simulink model "Vehicle_model_with_controllers_in_continuous_system_V01"  (R2026a)
settings: Solver=VariableStepAuto  StopTime=inf  RelTol=1e-6
InitFcn:
  | run('Vehicle_parameters_values_V1_MIL.m')
undefined symbols (not defined in the file): Finaldrive, Transmission, Vehicle
libraries: slpidlib x2
(part 1 of 2)
settings Model: PacingRate=0.500000  Creator=irfan  LastModifiedBy=irfan
settings SolverCC: ShapePreserveControl=EnableAll  ZeroCrossControl=EnableAll  ZeroCrossAlgorithm=Adaptive  MinimalZcImpactIntegration=on
settings DebuggingCC: ReadBeforeWriteMsg=DisableAll  WriteAfterWriteMsg=DisableAll  WriteAfterReadMsg=DisableAll  MultiTaskDSMMsg=none
settings SFSimCC: SFSimEcho=off

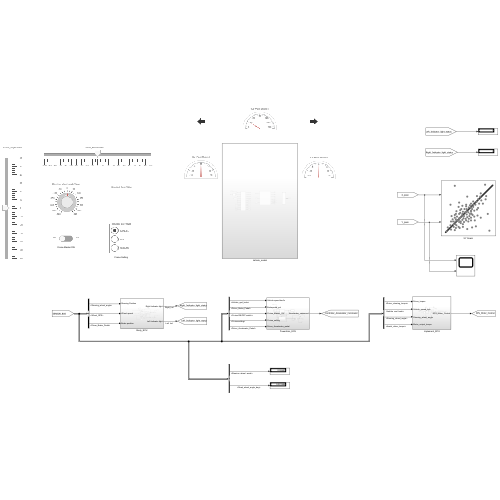
[thumbnail: Simulink's stored preview of the top-level diagram]
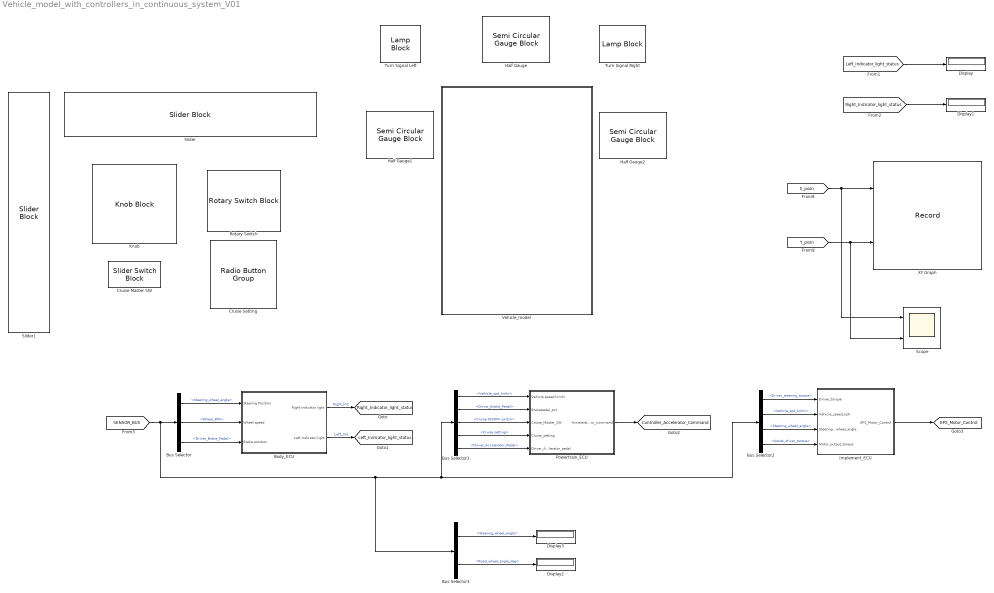
== system Vehicle_model_with_controllers_in_continuous_system_V01 ==
  Body_ECU : Subsystem
  Bus Selector : BusSelector  OutputSignals=Steering_wheel_angle,Wheel_RPS,Driver_Brake_Pedal
  Bus Selector1 : BusSelector  OutputSignals=Vehicle_spd_kmhr,Driver_Brake_Pedal,Cruise ON/OFF switch,Cruise setting,Driver_Accelerator_Pedal
  Bus Selector2 : BusSelector  OutputSignals=Driver_steering_torque,Vehicle_spd_kmhr,Steering_wheel_angle,Assist_driver_torque
  Bus Selector3 : BusSelector  OutputSignals=Steering_wheel_angle,Road_wheel_angle_deg
  Cruise Master SW : SliderSwitchBlock  LabelPosition=Hide
  Cruise Setting : RadioButtonGroup  LabelPosition=Hide  SelectedLabel=CANCEL  ButtonGroupName=CRUISE_SETTING
  Display{,1..3} (4 alike) : Display
  Half Gauge : SemiCircularGaugeBlock  ScaleMax=180  FontColor=[0.0, 0.0, 0.0]
  Half Gauge1 : SemiCircularGaugeBlock  ScaleMin=-15  ScaleMax=15  TickInterval=5  FontColor=[0.0, 0.0, 0.0]
  Half Gauge2 : SemiCircularGaugeBlock  ScaleMin=-15  ScaleMax=15  TickInterval=5  FontColor=[0.0, 0.0, 0.0]
  Implement_ECU : Subsystem
  Knob : KnobBlock  ScaleMin=-540  ScaleMax=540  TickInterval=90
  Powertrain_ECU : Subsystem
  Rotary Switch : RotarySwitchBlock
  Scope : Scope  NumInputPorts=2
      settings: ActiveDisplayYMinimum=-16.839005262411046  ActiveDisplayYMaximum=22.945762776973872  DataLoggingVariableName=ScopeData55
  Slider : SliderBlock  ScaleMin=-100  TickInterval=10
  Slider1 : SliderBlock  ScaleMin=-60  ScaleMax=60  TickInterval=10
  Turn Signal Left : LampBlock  LabelPosition=Hide  DefaultColor=[192.0, 192.0, 192.0]  Icon=TurnSignalLeft
  Turn Signal Right : LampBlock  LabelPosition=Hide  DefaultColor=[192.0, 192.0, 192.0]  Icon=TurnSignalRight
  Vehicle_model : Subsystem
  XY Graph : Record  NumPorts=2.0  FileSettingsInternal="{\"entries\":[{\"content\":{\"excelSettings\":{\"content\":{},\"type\":\"Streamout.ExcelSettings\"},\"parquetSettings\":{\"content\":{},\"type\":\"Streamout.ParquetSettings\"}},\"type\":\"Streamout.FileSettingStorage\",\"uuid\":\"\"}],\"packageUris\":[\"http:\\/\\/schema.mathworks.com\\/mf0\\/streamout_blocks\\/R2020a\"],\"version\":\"1.0\"}"  FrameSettings=[0, 0]  Layout=[1 1]  SignalsInternal="{\"entries\":[{\"content\":{\"signals\":[{\"content\":{\"blockPath\":[],\"dimensions\":[1],\"domain\":\"\",\"lineColor\":\"#a2142f\",\"plots\":[ 1 ],\"port\":1,\"sid\":[\"\"],\"signalID\":1,\"signalName\":\"From8\"},\"type\":\"RecordBlkView.Signal\",\"uuid\":\"\"},{\"content\":{\"blockPath\":[],\"dimensions\":[1],\"domain\":\"\",\"lineColor\":\"#139fff\",\"plots\":[ 1 ],\"port\":2,\"sid\":[\"\"],\"signalID\":2,\"signalName\":\"From9\"},\"type\":\"RecordBlkView.Signal\",\"uuid\":\"\"},{\"content\":{\"blockPath\":[],\"dimensions\":[1],\"domain\":\"\",\"lineColor\":\"#77ac30\",\"lineWidth\":2,\"sid\":[\"\"],\"signalID\":3,\"signalName\":\"Grade_angle:Value\"},\"type\":\"RecordBlkView.Signal\",\"uuid\":\"\"},{\"content\":{\"blockPath\":[],\"dimensions\":[1],\"domain\":\"\",\"lineColor\":\"#4dbeee\",\"lineWidth\":2,\"sid\":[\"\"],\"signalID\":4,\"signalName\":\"CruiseMasterSW:Value\"},\"type\":\"RecordBlkView.Signal\",\"uuid\":\"\"},{\"content\":{\"blockPath\":[],\"dimensions\":[1],\"domain\":\"\",\"lineColor\":\"#a2142f\",\"lineWidth\":2,\"sid\":[\"\"],\"signalID\":5,\"signalName\":\"Cruisesetting:Value\"},\"type\":\"RecordBlkView.Signal\",\"uuid\":\"\"},{\"content\":{\"blockPath\":[],\"dimensions\":[1],\"domain\":\"\",\"lineColor\":\"#139fff\",\"lineWidth\":2,\"sid\":[\"\"],\"signalID\":6,\"signalName\":\"Driver_Pedal:Value\"},\"type\":\"RecordBlkView.Signal\",\"uuid\":\"\"},{\"content\":{\"blockPath\":[],\"dimensions\":[1],\"domain\":\"\",\"lineColor\":\"#ff6929\",\"lineWidth\":2,\"sid\":[\"\"],\"signalID\":7,\"signalName\":\"Selected_Gear:Value\"},\"type\":\"RecordBlkView.Signal\",\"uuid\":\"\"},{\"content\":{\"blockPath\":[],\"dimensions\":[1],\"domain\":\"\",\"lineColor\":\"#b746ff\",\"lineWidth\":2,\"sid\":[\"\"],\"signalID\":8,\"signalName\":\"Steering_wheel_angle:Value\"},\"type\":\"RecordBlkView.Signal\",\"uuid\":\"\"}]},\"type\":\"RecordBlkView.InputSignals\",\"uuid\":\"\"}],\"packageUris\":[\"http:\\/\\/schema.mathworks.com\\/mf0\\/streamout_blocks\\/R2020a\"],\"version\":\"1.0\"}"  VisualizationBindings="{\"xyplotplugin\":{\"info\":[{\"series\":[{\"bindingParametersList\":[{\"parameter\":\"X-Axis\",\"signalID\":1,\"signalName\":\"From8\"},{\"parameter\":\"Y-Axis\",\"signalID\":2,\"signalName\":\"From9\"}],\"seriesID\":0}],\"subplotID\":1}]}}"  CompatibilityTag=XY
  tag scope: Controller_Accelerator_Command=global, EPS_Motor_Control=global, Left_Indicator_light_status=global, Right_Indicator_light_status=global
  wires:
  Bus Selector/1 -> Body_ECU/1(Steering Position)  "<Steering_wheel_angle>"
  Bus Selector/3 -> Body_ECU/3(Brake position)  "<Driver_Brake_Pedal>"
  Body_ECU/1(Right Indicator light) -> [Right_Indicator_light_status]  "Right_Ind"
  Body_ECU/2(Left Indicator light) -> [Left_Indicator_light_status]  "Left_Ind"
  Bus Selector/2 -> Body_ECU/2(Wheel speed)  "<Wheel_RPS>"
  Bus Selector1/1 -> Powertrain_ECU/1(Vehicle speed km/hr)  "<Vehicle_spd_kmhr>"
  Bus Selector1/2 -> Powertrain_ECU/2(Brakepedal_pct)  "<Driver_Brake_Pedal>"
  Bus Selector1/3 -> Powertrain_ECU/3(Cruise_Master_SW)  "<Cruise ON/OFF switch>"
  Bus Selector1/4 -> Powertrain_ECU/4(Cruise_setting)  "<Cruise setting>"
  Bus Selector1/5 -> Powertrain_ECU/5(Driver_Accelerator_pedal)  "<Driver_Accelerator_Pedal>"
  Powertrain_ECU/1(Accelerator_command) -> [Controller_Accelerator_Command]
  Bus Selector2/1 -> Implement_ECU/1(Driver_torque)  "<Driver_steering_torque>"
  Bus Selector2/2 -> Implement_ECU/2(Vehicle_speed_kph)  "<Vehicle_spd_kmhr>"
  Bus Selector2/3 -> Implement_ECU/3(Steering_wheel_angle)  "<Steering_wheel_angle>"
  Bus Selector2/4 -> Implement_ECU/4(Motor_output_torque)  "<Assist_driver_torque>"
  Implement_ECU/1(EPS_Motor_Control) -> [EPS_Motor_Control]
  [X_posn] -> Scope/1, XY Graph/1
  [Y_posn] -> Scope/2, XY Graph/2
  [Left_Indicator_light_status] -> Display/1
  [Right_Indicator_light_status] -> Display1/1
  [SENSOR_BUS] -> Bus Selector3/1, Bus Selector2/1, Bus Selector1/1, Bus Selector/1
  Bus Selector3/2 -> Display2/1  "<Road_wheel_angle_deg>"
  Bus Selector3/1 -> Display3/1  "<Steering_wheel_angle>"

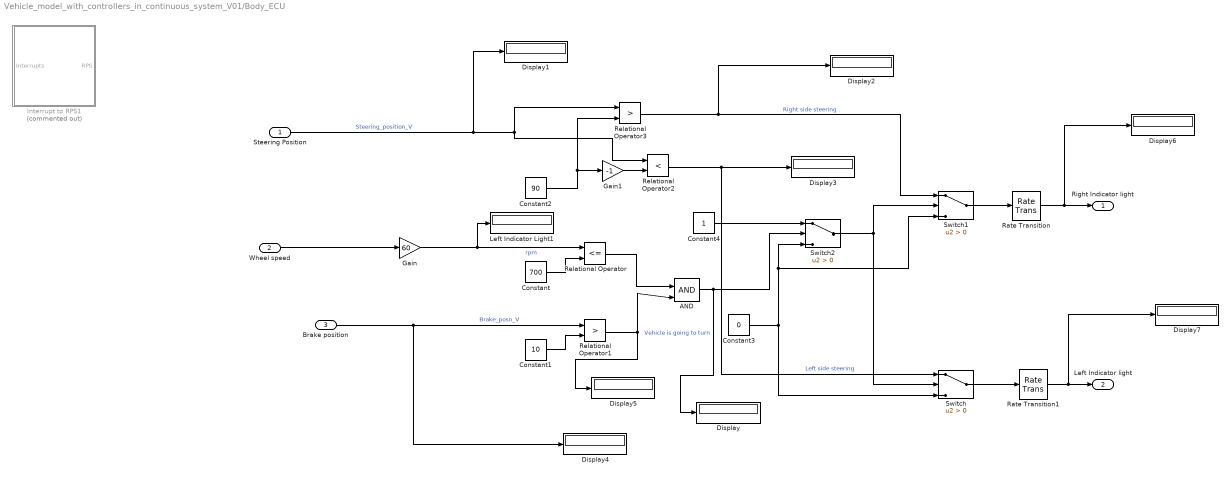
== system Vehicle_model_with_controllers_in_continuous_system_V01/Body_ECU ==
  Steering Position : Inport  OutDataTypeStr=single  PortDimensions=1
  Wheel speed : Inport  Port=2  OutDataTypeStr=double  PortDimensions=1
  Brake position : Inport  Port=3  OutDataTypeStr=double  PortDimensions=1
  AND : Logic  IconShape=distinctive  AllPortsSameDT=off  OutDataTypeStr=boolean
  Constant : Constant  Value=700
  Constant1 : Constant  Value=10
  Constant2 : Constant  Value=90
  Constant3 : Constant  Value=0
  Constant4 : Constant
  Display{,1..7} (8 alike) : Display
  Gain : Gain  Gain=60
  Gain1 : Gain  Gain=-1
  Interrupt to RPS1 : Subsystem  Commented=on
  Left Indicator Light1 : Display
  Rate Transition : RateTransition
  Rate Transition1 : RateTransition
  Relational Operator : RelationalOperator  Operator=<=  OutDataTypeStr=boolean  RndMeth=Simplest  InputSameDT=off
  Relational Operator1 : RelationalOperator  Operator=>  OutDataTypeStr=boolean  RndMeth=Simplest  InputSameDT=off
  Relational Operator2 : RelationalOperator  Operator=<  OutDataTypeStr=boolean  RndMeth=Simplest  InputSameDT=off
  Relational Operator3 : RelationalOperator  Operator=>  OutDataTypeStr=boolean  RndMeth=Simplest  InputSameDT=off
  Switch : Switch  Criteria=u2 > Threshold  SaturateOnIntegerOverflow=off  InputSameDT=off
  Switch1 : Switch  Criteria=u2 > Threshold  SaturateOnIntegerOverflow=off  InputSameDT=off
  Switch2 : Switch  Criteria=u2 > Threshold  SaturateOnIntegerOverflow=off  InputSameDT=off
  Right Indicator light : Outport  OutDataTypeStr=double  PortDimensions=1  SampleTime=[0,1]
  Left Indicator light : Outport  Port=2  OutDataTypeStr=double  PortDimensions=1  SampleTime=[0,1]
  wires:
  Rate Transition1/1 -> Display7/1, Left Indicator light/1
  Relational Operator/1 -> AND/1
  Rate Transition/1 -> Display6/1, Right Indicator light/1
  Constant1/1 -> Relational Operator1/2
  Constant4/1 -> Switch2/1
  Gain/1 -> Relational Operator/1, Left Indicator Light1/1  "rpm"
  Switch2/1 -> Switch/2, Switch1/2
  Constant/1 -> Relational Operator/2
  AND/1 -> Display/1, Switch2/2  "Vehicle is going to turn"
  Switch/1 -> Rate Transition1/1
  Constant2/1 -> Gain1/1, Relational Operator3/2
  Relational Operator1/1 -> AND/2, Display5/1
  Steering Position/1 -> Display1/1, Relational Operator3/1, Relational Operator2/1  "Steering_position_V"
  Brake position/1 -> Display4/1, Relational Operator1/1  "Brake_posn_V"
  Constant3/1 -> Switch/3, Switch1/3, Switch2/3
  Relational Operator2/1 -> Switch/1, Display3/1  "Left side steering"
  Relational Operator3/1 -> Display2/1, Switch1/1  "Right side steering"
  Switch1/1 -> Rate Transition/1
  Gain1/1 -> Relational Operator2/2
  Wheel speed/1 -> Gain/1

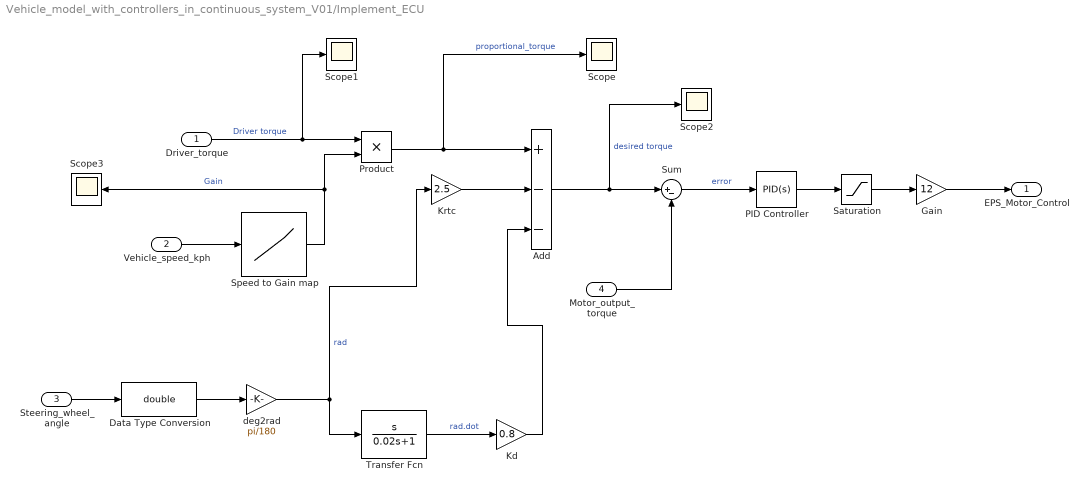
== system Vehicle_model_with_controllers_in_continuous_system_V01/Implement_ECU ==
  Driver_torque : Inport
  Vehicle_speed_kph : Inport  Port=2
  Steering_wheel_angle : Inport  Port=3
  Motor_output_torque : Inport  Port=4
  Add : Sum  Inputs=+--
  Data Type Conversion : DataTypeConversion  OutDataTypeStr=double  SaturateOnIntegerOverflow=off  RndMeth=Floor
  Gain : Gain  Gain=12
  Kd : Gain  Gain=0.8
  Krtc : Gain  Gain=2.5
  PID Controller : slpidlib/PID Controller  Controller=PID  Form=Parallel  TimeDomain=Continuous-time  UseExternalTs=off  SampleTime=-1  IntegratorMethod=Forward Euler  FilterMethod=Forward Euler  ControllerParametersSource=internal  P=1  I=5  UseKiTs=off  D=0  UseExternalDerivativeSource=off  N=100  UseFilter=on  TunerSelectOption=Transfer Function Based (PID Tuner App)  InitialConditionSource=internal  InitialConditionForIntegrator=0  InitialConditionForFilter=0  DifferentiatorICPrevScaledInput=0  ExternalReset=none  TrackingMode=off  Kt=1  LimitOutput=off  SatLimitsSource=internal  UpperSaturationLimit=inf  LowerSaturationLimit=-inf  LinearizeAsGain=on  AntiWindupMode=none  Kb=1  LimitIntegrator=off  UpperIntegratorSaturationLimit=inf  LowerIntegratorSaturationLimit=-inf  POutMin=[]  POutMax=[]  IOutMin=[]  IOutMax=[]  DOutMin=[]  DOutMax=[]  NOutMin=[]  NOutMax=[]  SumOutMin=[]  SumOutMax=[]  SaturationOutMin=[]  SaturationOutMax=[]  PParamMin=[]  PParamMax=[]  IParamMin=[]  IParamMax=[]  DParamMin=[]  DParamMax=[]  NParamMin=[]  NParamMax=[]  KbParamMin=[]  KbParamMax=[]  KtParamMin=[]  KtParamMax=[]  KbOutMin=[]  KbOutMax=[]  KtOutMin=[]  KtOutMax=[]  IntegratorOutMin=[]  IntegratorOutMax=[]  FilterOutMin=[]  FilterOutMax=[]  SumI1OutMin=[]  SumI1OutMax=[]  SumI2OutMin=[]  SumI2OutMax=[]  SumI3OutMin=[]  SumI3OutMax=[]  SumI4OutMin=[]  SumI4OutMax=[]  SumDOutMin=[]  SumDOutMax=[]  DifferentiatorOutMin=[]  DifferentiatorOutMax=[]  FilterDiffOutCoefMin=[]  FilterDiffOutCoefMax=[]  ReciprocalOutMin=[]  ReciprocalOutMax=[]  SumDenOutMin=[]  SumDenOutMax=[]  SumNumOutMin=[]  SumNumOutMax=[]  DivideOutMin=[]  DivideOutMax=[]  UdiffTsProdOutMin=[]  UdiffTsProdOutMax=[]  NTsProdOutMin=[]  NTsProdOutMax=[]  UintegralTsProdOutMin=[]  UintegralTsProdOutMax=[]  UngainTsProdOutMin=[]  UngainTsProdOutMax=[]  ClampingZeroOutDataTypeStr=Inherit: Inherit via back propagation  ClampingZeroOutMin=[]  ClampingZeroOutMax=[]  FilterDenConstantOutDataTypeStr=Inherit: Inherit via back propagation  FilterDenConstantOutMin=[]  FilterDenConstantOutMax=[]  PCopyOutDataTypeStr=Inherit: Inherit via back propagation  PCopyOutMin=[]  PCopyOutMax=[]  NCopyOutDataTypeStr=Inherit: Inherit via back propagation  NCopyOutMin=[]  NCopyOutMax=[]  IntegratorContinuousStateAttributes=''  IntegratorStateMustResolveToSignalObject=off  IntegratorRTWStateStorageClass=Auto  FilterContinuousStateAttributes=''  FilterStateMustResolveToSignalObject=off  FilterRTWStateStorageClass=Auto  ParallelPVariant=InternalParameters  IdealPVariant=Disabled  IVariant=InternalParameters  DVariant=InternalParameters  IntegratorVariant=Continuous  SatVariant=Disabled  AWVariant=Passthrough  PCopyVariant=Disabled  TRVariant=Disabled  FdbkBlocksVariant=Forward  IdealPFdbkVariant=Disabled  SatFdbkVariant=Disabled  DerivativeFilterVariant=ContFilter  NVariant=InternalParameters  NCopyVariant=Disabled  FilterICVariant=InternalICsFilter  IntegratorICVariant=InternalICs  ExternalResetVariant=Disabled  TRSumVariant=Passthrough  SumFdbkVariant=Disabled  SumVariant=Sum_PID  TsampFilterVariant=InternalTs  TsampNgainVariant=Passthrough  TsampIntegralVariant=Disabled_SignalSpec  ExternalSaturationOutDataTypeStr=Inherit: Same as second input  DerivativeSourceVariant=ErrorSignal  PreIntVariant=InternalPreInt
  Product : Product
  Saturation : Saturate  UpperLimit=1  LowerLimit=0
  Scope{,1..3} (4 alike) : Scope
      Scope settings: DataLoggingVariableName=ScopeData9
      Scope1 settings: ActiveDisplayYMinimum=33.050124587675704  ActiveDisplayYMaximum=33.050574191834883  DataLoggingVariableName=ScopeData10
      Scope2 settings: ActiveDisplayYMinimum=13.852646360753944  ActiveDisplayYMaximum=13.860007449671043  DataLoggingVariableName=ScopeData11
      Scope3 settings: ActiveDisplayYMinimum=-1  ActiveDisplayYMaximum=1  DataLoggingVariableName=ScopeData12
  Speed to Gain map : Lookup_n-D  NumberOfTableDimensions=1  BreakpointsForDimension1=Vehicle.speedvalues  Table=Vehicle.torquegains  InternalRulePriority=Speed  RndMeth=Simplest
  Sum : Sum  Inputs=|+-
  Transfer Fcn : TransferFcn  Numerator=[1 0]  Denominator=[0.02 1]
  deg2rad : Gain  Gain=pi/180
  EPS_Motor_Control : Outport
  wires:
  Speed to Gain map/1 -> Product/2, Scope3/1  "Gain"
  Sum/1 -> PID Controller/1  "error"
  Product/1 -> Scope/1, Add/1  "proportional_torque"
  Driver_torque/1 -> Scope1/1, Product/1  "Driver torque"
  Vehicle_speed_kph/1 -> Speed to Gain map/1
  PID Controller/1 -> Saturation/1
  Motor_output_torque/1 -> Sum/2
  Saturation/1 -> Gain/1
  Gain/1 -> EPS_Motor_Control/1
  Krtc/1 -> Add/2
  Steering_wheel_angle/1 -> Data Type Conversion/1
  deg2rad/1 -> Transfer Fcn/1, Krtc/1  "rad"
  Transfer Fcn/1 -> Kd/1  "rad.dot"
  Add/1 -> Scope2/1, Sum/1  "desired torque"
  Kd/1 -> Add/3
  Data Type Conversion/1 -> deg2rad/1

== system Vehicle_model_with_controllers_in_continuous_system_V01/Powertrain_ECU ==
  Vehicle speed km/hr : Inport
  Brakepedal_pct : Inport  Port=2
  Cruise_Master_SW : Inport  Port=3
  Cruise_setting : Inport  Port=4
  Driver_Accelerator_pedal : Inport  Port=5
  Chart : Stateflow chart  TreatAsAtomicUnit=on
  Display : Display
  Display1 : Display
  Display2 : Display
  Enabled Subsystem : Subsystem  TreatAsAtomicUnit=on
  Scope : Scope
      settings: ActiveDisplayYMinimum=-1  ActiveDisplayYMaximum=1  DataLoggingVariableName=ScopeData6
  Scope1 : Scope
      settings: ActiveDisplayYMinimum=-5.6388294949677089  ActiveDisplayYMaximum=36.997696709911374  DataLoggingVariableName=ScopeData7
  Switch : Switch  Criteria=u2 > Threshold  SaturateOnIntegerOverflow=off  InputSameDT=off
  Accelerator_command : Outport
  wires:
  Chart/1(Set_spd) -> Enabled Subsystem/2(Set_spd), Display/1
  Vehicle speed km/hr/1 -> Chart/3(Vehicle_spd), Enabled Subsystem/1(Vehicle speed km/hr)
  Cruise_Master_SW/1 -> Chart/4(Cruise_Master_SW)
  Brakepedal_pct/1 -> Chart/2(Brk_pdl)
  Enabled Subsystem/1(CruiseAccelPedal_pct) -> Scope/1, Switch/1
  Cruise_setting/1 -> Chart/1(Cr_St)
  Chart/2(Cruise_enable) -> Display1/1, Enabled Subsystem/Enable, Enabled Subsystem/3(CruiseEnable), Switch/2
  Driver_Accelerator_pedal/1 -> Switch/3
  Switch/1 -> Scope1/1, Display2/1, Accelerator_command/1

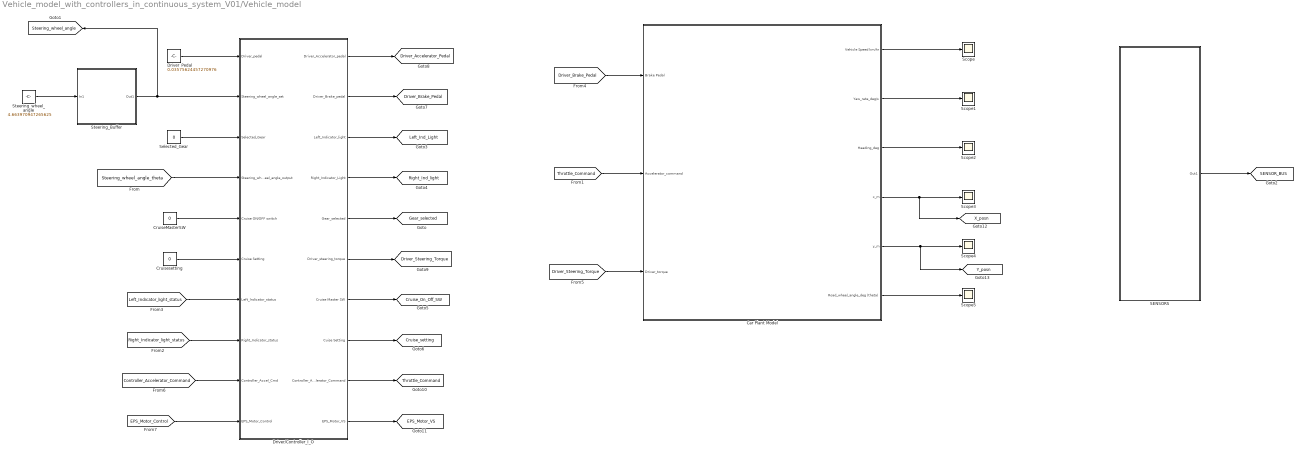
== system Vehicle_model_with_controllers_in_continuous_system_V01/Vehicle_model ==
  Car Plant Model : Subsystem
  CruiseMasterSW : Constant  Value=0
  Cruisesetting : Constant  Value=0
  Driver/Controller_I_O : Subsystem
  Driver_Pedal : Constant  Value=0.03575624457270976
  SENSORS : Subsystem
  Scope{,1..5} (6 alike) : Scope
      Scope settings: ActiveDisplayYMinimum=52.703316874102136  ActiveDisplayYMaximum=58.921674606812623
      Scope2 settings: DataLoggingVariableName=ScopeData2
      Scope3 settings: DataLoggingVariableName=ScopeData3
      Scope4 settings: DataLoggingVariableName=ScopeData4
      Scope5 settings: ActiveDisplayYMinimum=-229.29250394050729  ActiveDisplayYMaximum=178.246522265426  DataLoggingVariableName=ScopeData5
  Selected_Gear : Constant  Value=0
  Steering_Buffer : Subsystem
  Steering_wheel_angle : Constant  Value=4.663970947265625
  tag scope: Cruise_On_Off_SW=global, Cruise_setting=global, Driver_Accelerator_Pedal=global, Driver_Brake_Pedal=global, Driver_Steering_Torque=global, EPS_Motor_VS=global, Gear_selected=global, Left_Ind_Light=global, Right_Ind_light=global, SENSOR_BUS=global, Steering_wheel_angle=global, Throttle_Command=global, X_posn=global, Y_posn=global
  wires:
  Selected_Gear/1 -> Driver/Controller_I_O/3(Selected_Gear)
  Driver_Pedal/1 -> Driver/Controller_I_O/1(Driver_pedal)
  [Steering_wheel_angle_theta] -> Driver/Controller_I_O/4(Steering_wheel_angle_output)
  Driver/Controller_I_O/5(Gear_selected) -> [Gear_selected]
  SENSORS/1(Out1) -> [SENSOR_BUS]
  Driver/Controller_I_O/3(Left_Indicator_light) -> [Left_Ind_Light]
  Driver/Controller_I_O/4(Right_Indicator_Light) -> [Right_Ind_light]
  Cruisesetting/1 -> Driver/Controller_I_O/6(Cruise Setting)
  CruiseMasterSW/1 -> Driver/Controller_I_O/5(Cruise ON/OFF switch)
  Car Plant Model/1(Vehicle Speed km/hr) -> Scope/1
  Car Plant Model/2(Yaw_rate_deg/s) -> Scope1/1
  Car Plant Model/3(Heading_deg) -> Scope2/1
  Car Plant Model/4(x_m) -> [X_posn], Scope3/1
  Car Plant Model/5(y_m) -> [Y_posn], Scope4/1
  Car Plant Model/6(Road_wheel_angle_deg (theta)) -> Scope5/1
  [Right_Indicator_light_status] -> Driver/Controller_I_O/8(Right_Indicator_status)
  [Left_Indicator_light_status] -> Driver/Controller_I_O/7(Left_lndicator_status)
  Driver/Controller_I_O/7(Cruise Master SW) -> [Cruise_On_Off_SW]
  Driver/Controller_I_O/8(Cuise Setting) -> [Cruise_setting]
  Driver/Controller_I_O/2(Driver_Brake_pedal) -> [Driver_Brake_Pedal]
  [Driver_Brake_Pedal] -> Car Plant Model/1(Brake Pedal)
  Driver/Controller_I_O/1(Driver_Accelerator_pedal) -> [Driver_Accelerator_Pedal]
  Driver/Controller_I_O/6(Driver_steering_torque) -> [Driver_Steering_Torque]
  [Driver_Steering_Torque] -> Car Plant Model/3(Driver_torque)
  [Controller_Accelerator_Command] -> Driver/Controller_I_O/9(Controller_Accel_Cmd)
  Driver/Controller_I_O/9(Controller_Accelerator_Command) -> [Throttle_Command]
  [EPS_Motor_Control] -> Driver/Controller_I_O/10(EPS_Motor_Control)
  Driver/Controller_I_O/10(EPS_Motor_VS) -> [EPS_Motor_VS]
  [Throttle_Command] -> Car Plant Model/2(Accelerator_command)
  Steering_wheel_angle/1 -> Steering_Buffer/1(In1)
  Steering_Buffer/1(Out1) -> [Steering_wheel_angle], Driver/Controller_I_O/2(Steering_wheel_angle_set)

== system Vehicle_model_with_controllers_in_continuous_system_V01/Body_ECU/Interrupt to RPS1 ==
  Interrupts : Inport
  Data Store Memory : DataStoreMemory  DataStoreName=Count  WriteAfterWriteMsg=warning  ShowAdditionalParam=off
  Pulse Generator : DiscretePulseGenerator  PulseType=Time based  Period=1.1  PulseWidth=10
  Scope3 : Scope
      settings: ActiveDisplayYMinimum=-0.12499999999999997  ActiveDisplayYMaximum=1.125  DataLoggingVariableName=ScopeData2
  Triggered Subsystem : Subsystem  TreatAsAtomicUnit=on
  Triggered Subsystem1 : Subsystem  TreatAsAtomicUnit=on
  RPS : Outport
  wires:
  Interrupts/1 -> Triggered Subsystem/Trigger
  Pulse Generator/1 -> Scope3/1, Triggered Subsystem1/Trigger
  Triggered Subsystem/1(RPS) -> RPS/1

== system Vehicle_model_with_controllers_in_continuous_system_V01/Powertrain_ECU/Enabled Subsystem ==
  Vehicle speed km/hr : Inport
  Set_spd : Inport  Port=2
  CruiseEnable : Inport  Port=3
  Enable : EnablePort  StatesWhenEnabling=reset
  Dead Zone : DeadZone
  NOT : Logic  Operator=NOT  IconShape=distinctive  AllPortsSameDT=off  OutDataTypeStr=boolean
  PID Controller : slpidlib/PID Controller  Controller=PID  Form=Parallel  TimeDomain=Continuous-time  UseExternalTs=off  SampleTime=-1  IntegratorMethod=Forward Euler  FilterMethod=Forward Euler  ControllerParametersSource=internal  P=1  I=0.5  UseKiTs=off  D=0  UseExternalDerivativeSource=off  N=100  UseFilter=on  TunerSelectOption=Transfer Function Based (PID Tuner App)  InitialConditionSource=internal  InitialConditionForIntegrator=0  InitialConditionForFilter=0  DifferentiatorICPrevScaledInput=0  ExternalReset=rising  TrackingMode=off  Kt=1  LimitOutput=on  SatLimitsSource=internal  UpperSaturationLimit=100  LowerSaturationLimit=0  LinearizeAsGain=on  AntiWindupMode=back-calculation  Kb=1  LimitIntegrator=off  UpperIntegratorSaturationLimit=inf  LowerIntegratorSaturationLimit=-inf  POutMin=[]  POutMax=[]  IOutMin=[]  IOutMax=[]  DOutMin=[]  DOutMax=[]  NOutMin=[]  NOutMax=[]  SumOutMin=[]  SumOutMax=[]  SaturationOutMin=[]  SaturationOutMax=[]  PParamMin=[]  PParamMax=[]  IParamMin=[]  IParamMax=[]  DParamMin=[]  DParamMax=[]  NParamMin=[]  NParamMax=[]  KbParamMin=[]  KbParamMax=[]  KtParamMin=[]  KtParamMax=[]  KbOutMin=[]  KbOutMax=[]  KtOutMin=[]  KtOutMax=[]  IntegratorOutMin=[]  IntegratorOutMax=[]  FilterOutMin=[]  FilterOutMax=[]  SumI1OutMin=[]  SumI1OutMax=[]  SumI2OutMin=[]  SumI2OutMax=[]  SumI3OutMin=[]  SumI3OutMax=[]  SumI4OutMin=[]  SumI4OutMax=[]  SumDOutMin=[]  SumDOutMax=[]  DifferentiatorOutMin=[]  DifferentiatorOutMax=[]  FilterDiffOutCoefMin=[]  FilterDiffOutCoefMax=[]  ReciprocalOutMin=[]  ReciprocalOutMax=[]  SumDenOutMin=[]  SumDenOutMax=[]  SumNumOutMin=[]  SumNumOutMax=[]  DivideOutMin=[]  DivideOutMax=[]  UdiffTsProdOutMin=[]  UdiffTsProdOutMax=[]  NTsProdOutMin=[]  NTsProdOutMax=[]  UintegralTsProdOutMin=[]  UintegralTsProdOutMax=[]  UngainTsProdOutMin=[]  UngainTsProdOutMax=[]  ClampingZeroOutDataTypeStr=Inherit: Inherit via back propagation  ClampingZeroOutMin=[]  ClampingZeroOutMax=[]  FilterDenConstantOutDataTypeStr=Inherit: Inherit via back propagation  FilterDenConstantOutMin=[]  FilterDenConstantOutMax=[]  PCopyOutDataTypeStr=Inherit: Inherit via back propagation  PCopyOutMin=[]  PCopyOutMax=[]  NCopyOutDataTypeStr=Inherit: Inherit via back propagation  NCopyOutMin=[]  NCopyOutMax=[]  IntegratorContinuousStateAttributes=''  IntegratorStateMustResolveToSignalObject=off  IntegratorRTWStateStorageClass=Auto  FilterContinuousStateAttributes=''  FilterStateMustResolveToSignalObject=off  FilterRTWStateStorageClass=Auto  ParallelPVariant=InternalParameters  IdealPVariant=Disabled  IVariant=InternalParameters  DVariant=InternalParameters  IntegratorVariant=Continuous  SatVariant=Enabled  AWVariant=BackCalculation  PCopyVariant=Disabled  TRVariant=Disabled  FdbkBlocksVariant=Forward  IdealPFdbkVariant=Disabled  SatFdbkVariant=Disabled  DerivativeFilterVariant=ContFilter  NVariant=InternalParameters  NCopyVariant=Disabled  FilterICVariant=InternalICsFilter  IntegratorICVariant=InternalICs  ExternalResetVariant=ExternalReset  TRSumVariant=Passthrough  SumFdbkVariant=Disabled  SumVariant=Sum_PID  TsampFilterVariant=InternalTs  TsampNgainVariant=Passthrough  TsampIntegralVariant=Disabled_SignalSpec  ExternalSaturationOutDataTypeStr=Inherit: Same as second input  DerivativeSourceVariant=ErrorSignal  PreIntVariant=InternalPreInt
  Rate Limiter : RateLimiter  RisingSlewLimit=25  FallingSlewLimit=-40  SampleTimeMode=inherited
  Saturation : Saturate  UpperLimit=100  LowerLimit=0
  Sum : Sum  Inputs=|+-
  CruiseAccelPedal_pct : Outport
  wires:
  Sum/1 -> Dead Zone/1
  Saturation/1 -> Rate Limiter/1
  CruiseEnable/1 -> NOT/1
  NOT/1 -> PID Controller/2
  Vehicle speed km/hr/1 -> Sum/2
  Set_spd/1 -> Sum/1
  PID Controller/1 -> Saturation/1
  Rate Limiter/1 -> CruiseAccelPedal_pct/1
  Dead Zone/1 -> PID Controller/1

== system Vehicle_model_with_controllers_in_continuous_system_V01/Vehicle_model/Car Plant Model ==
  Brake Pedal : Inport
  Accelerator_command : Inport  Port=2
  Driver_torque : Inport  Port=3
  Display : Display
  Display1 : Display
  "Electrical " : Subsystem
  Engine : Subsystem
  Grade_angle : Constant  Value=0.2070750647109634
  Transmission : Subsystem
  Vehicle Dynamics : Subsystem
  Vehicle Speed km/hr : Outport
  Yaw_rate_deg/s : Outport  Port=2
  Heading_deg : Outport  Port=3
  x_m : Outport  Port=4
  y_m : Outport  Port=5
  Road_wheel_angle_deg (theta) : Outport  Port=6
  wires:
  Engine/1(Engine_Output_Torque) -> Transmission/1(Engine_torque)
  [Gear_selected] -> Transmission/2(Selected_Gear)
  Brake Pedal/1 -> Vehicle Dynamics/1(Brake Pedal)
  Transmission/1(Wheel_torque) -> Vehicle Dynamics/2(Wheel torque)
  Grade_angle/1 -> Vehicle Dynamics/3(Grade_angle_deg)
  Vehicle Dynamics/6(Road_wheel_angle_deg (theta)) -> Road_wheel_angle_deg (theta)/1
  Vehicle Dynamics/5(y_m) -> y_m/1
  Transmission/2(Engine_rpm) -> Engine/2(Engine_rpm)
  Accelerator_command/1 -> Engine/1(Throttle_command)
  Driver_torque/1 -> Vehicle Dynamics/4(Driver_torque)
  Vehicle Dynamics/1(Vehicle Speed km/hr) -> Vehicle Speed km/hr/1
  Vehicle Dynamics/4(x_m) -> x_m/1
  Vehicle Dynamics/3(Heading_deg) -> Heading_deg/1
  Vehicle Dynamics/2(Yaw_rate_deg/s) -> Yaw_rate_deg/s/1
  [Left_Ind_Light] -> "Electrical "/1(Left_Ind_Status)
  [Right_Ind_light] -> "Electrical "/2(Right_Ind_Status)
  "Electrical "/1(Left_Indicator_light) -> Display/1
  "Electrical "/2(Right_Indicator_Light) -> Display1/1

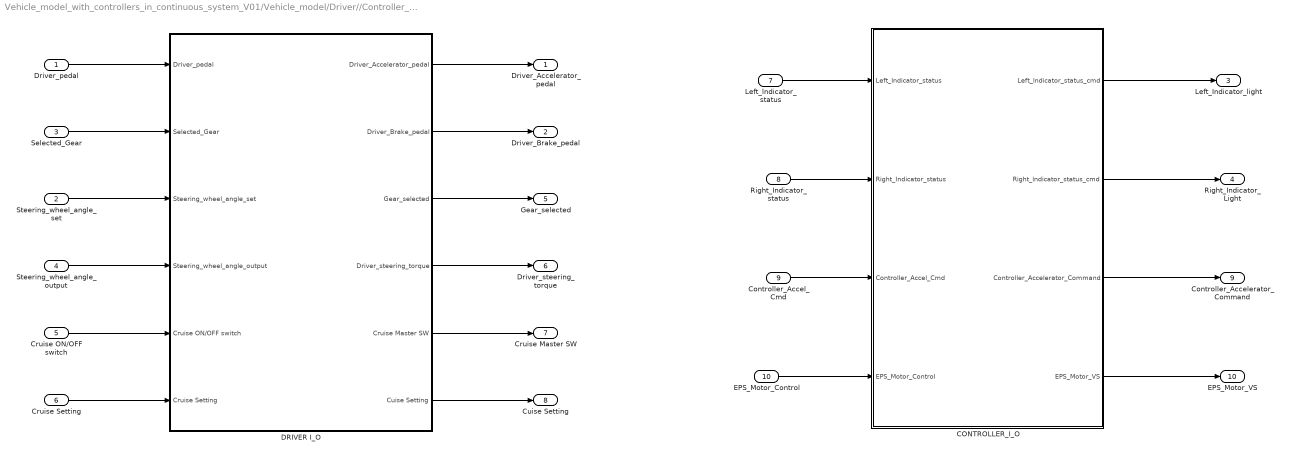
== system Vehicle_model_with_controllers_in_continuous_system_V01/Vehicle_model/Driver//Controller_I_O ==
  Driver_pedal : Inport
  Steering_wheel_angle_set : Inport  Port=2
  Selected_Gear : Inport  Port=3
  Steering_wheel_angle_output : Inport  Port=4
  Cruise ON/OFF switch : Inport  Port=5
  Cruise Setting : Inport  Port=6
  Left_lndicator_status : Inport  Port=7
  Right_Indicator_status : Inport  Port=8
  Controller_Accel_Cmd : Inport  Port=9
  EPS_Motor_Control : Inport  Port=10
  CONTROLLER_I_O : Subsystem
  DRIVER I_O : Subsystem
  Driver_Accelerator_pedal : Outport
  Driver_Brake_pedal : Outport  Port=2
  Left_Indicator_light : Outport  Port=3
  Right_Indicator_Light : Outport  Port=4
  Gear_selected : Outport  Port=5
  Driver_steering_torque : Outport  Port=6
  Cruise Master SW : Outport  Port=7
  Cuise Setting : Outport  Port=8
  Controller_Accelerator_Command : Outport  Port=9
  EPS_Motor_VS : Outport  Port=10
  wires:
  CONTROLLER_I_O/1(Left_lndicator_status_cmd) -> Left_Indicator_light/1
  CONTROLLER_I_O/2(Right_lndicator_status_cmd) -> Right_Indicator_Light/1
  Driver_pedal/1 -> DRIVER I_O/1(Driver_pedal)
  Selected_Gear/1 -> DRIVER I_O/2(Selected_Gear)
  Steering_wheel_angle_set/1 -> DRIVER I_O/3(Steering_wheel_angle_set)
  Steering_wheel_angle_output/1 -> DRIVER I_O/4(Steering_wheel_angle_output)
  Cruise ON/OFF switch/1 -> DRIVER I_O/5(Cruise ON/OFF switch)
  Cruise Setting/1 -> DRIVER I_O/6(Cruise Setting)
  DRIVER I_O/2(Driver_Brake_pedal) -> Driver_Brake_pedal/1
  DRIVER I_O/1(Driver_Accelerator_pedal) -> Driver_Accelerator_pedal/1
  DRIVER I_O/3(Gear_selected) -> Gear_selected/1
  DRIVER I_O/4(Driver_steering_torque) -> Driver_steering_torque/1
  DRIVER I_O/5(Cruise Master SW) -> Cruise Master SW/1
  DRIVER I_O/6(Cuise Setting) -> Cuise Setting/1
  Left_lndicator_status/1 -> CONTROLLER_I_O/1(Left_lndicator_status)
  Right_Indicator_status/1 -> CONTROLLER_I_O/2(Right_Indicator_status)
  Controller_Accel_Cmd/1 -> CONTROLLER_I_O/3(Controller_Accel_Cmd)
  CONTROLLER_I_O/3(Controller_Accelerator_Command) -> Controller_Accelerator_Command/1
  EPS_Motor_Control/1 -> CONTROLLER_I_O/4(EPS_Motor_Control)
  CONTROLLER_I_O/4(EPS_Motor_VS) -> EPS_Motor_VS/1

== system Vehicle_model_with_controllers_in_continuous_system_V01/Vehicle_model/SENSORS ==
  Bus Creator : BusCreator  Inputs=28
  DASHBOARD AND OTHER SENSORS/COMMUNICATION : Subsystem
  Data Type Conversion : DataTypeConversion  OutDataTypeStr=single  SaturateOnIntegerOverflow=off  RndMeth=Floor
  Data Type Conversion2 : DataTypeConversion  OutDataTypeStr=double  SaturateOnIntegerOverflow=off  RndMeth=Floor
  PEDAL SENSORS : Subsystem
  POWER TRAIN SENSORS : Subsystem
  STEERING : Subsystem
  VEHICLE MOTION SENSORS : Subsystem
  WHEEL SPEED SENSORS : Subsystem
  Out1 : Outport
  wires:
  POWER TRAIN SENSORS/2(Out2) -> Bus Creator/23  "Engine_output_torque"
  WHEEL SPEED SENSORS/2(Out2) -> Bus Creator/14  "Front_left_wheel_spd_mps"
  STEERING/5(Out5) -> Bus Creator/5  "Actual_steering_wheel_speed_degps"
  STEERING/1(Out1) -> Data Type Conversion/1  "Steering_wheel_angle"
  WHEEL SPEED SENSORS/1(Out1) -> Bus Creator/13  "Front_right_wheel_spd_mps"
  STEERING/2(Out2) -> Bus Creator/2  "Driver_steering_torque"
  STEERING/3(Out3) -> Bus Creator/3  "Road_wheel_angle_deg"
  POWER TRAIN SENSORS/1(Out1) -> Bus Creator/22  "Engine_RPM"
  WHEEL SPEED SENSORS/3(Out3) -> Bus Creator/15  "Rear_right_wheel_spd_mps"
  WHEEL SPEED SENSORS/7(Out7) -> Data Type Conversion2/1  "Wheel_RPS_Interrupts"
  STEERING/4(Out4) -> Bus Creator/4  "Assist_driver_torque"
  POWER TRAIN SENSORS/4(Out4) -> Bus Creator/25  "Wheel_Torque"
  PEDAL SENSORS/1(Out1) -> Bus Creator/20  "Driver_Accelerator_Pedal"
  WHEEL SPEED SENSORS/4(Out4) -> Bus Creator/16  "Rear_left_wheel_spd_mps"
  WHEEL SPEED SENSORS/5(Out5) -> Bus Creator/17  "Wheel_RPM"
  WHEEL SPEED SENSORS/6(Out6) -> Bus Creator/18  "Wheel_RPS"
  Data Type Conversion/1 -> Bus Creator/1  "Steering_wheel_angle"
  VEHICLE MOTION SENSORS/1(Out1) -> Bus Creator/6  "Vehicle_spd_kmhr"
  VEHICLE MOTION SENSORS/2(Out2) -> Bus Creator/7  "Vehicle_spd_mps"
  VEHICLE MOTION SENSORS/3(Out3) -> Bus Creator/8  "Longitudinal_acceleration_mps2"
  VEHICLE MOTION SENSORS/4(Out4) -> Bus Creator/9  "Yaw_rate_degps"
  VEHICLE MOTION SENSORS/5(Out5) -> Bus Creator/10  "Heading_deg"
  VEHICLE MOTION SENSORS/6(Out6) -> Bus Creator/11  "x_posn_m"
  VEHICLE MOTION SENSORS/7(Out7) -> Bus Creator/12  "y_posn_m"
  PEDAL SENSORS/2(Out2) -> Bus Creator/21  "Driver_Brake_Pedal"
  POWER TRAIN SENSORS/3(Out3) -> Bus Creator/24  "Selected_Gear"
  DASHBOARD AND OTHER SENSORS/COMMUNICATION/1(Out1) -> Bus Creator/26  "Cruise ON/OFF switch"
  DASHBOARD AND OTHER SENSORS/COMMUNICATION/2(Out2) -> Bus Creator/27  "Cruise setting"
  Bus Creator/1 -> Out1/1
  DASHBOARD AND OTHER SENSORS/COMMUNICATION/3(Out3) -> Bus Creator/28  "Gear_Selected"
  Data Type Conversion2/1 -> Bus Creator/19  "Wheel_RPS_Interrupts"

== system Vehicle_model_with_controllers_in_continuous_system_V01/Vehicle_model/Steering_Buffer ==
  In1 : Inport
  Constant1 : Constant  Value=90
  Gain : Gain  Gain=-1
  OR : Logic  Operator=OR  IconShape=distinctive  AllPortsSameDT=off  OutDataTypeStr=boolean
  Relational Operator : RelationalOperator  Operator=<  OutDataTypeStr=boolean  RndMeth=Simplest  InputSameDT=off
  Relational Operator1 : RelationalOperator  Operator=>  OutDataTypeStr=boolean  RndMeth=Simplest  InputSameDT=off
  Switch : Switch  Criteria=u2 > Threshold  SaturateOnIntegerOverflow=off  InputSameDT=off
  Zero : Constant  Value=0
  Out1 : Outport
  wires:
  Switch/1 -> Out1/1
  Constant1/1 -> Gain/1, Relational Operator1/2
  Zero/1 -> Switch/3
  Relational Operator1/1 -> OR/2
  Relational Operator/1 -> OR/1
  OR/1 -> Switch/2
  Gain/1 -> Relational Operator/2
  In1/1 -> Relational Operator1/1, Relational Operator/1, Switch/1

== system Vehicle_model_with_controllers_in_continuous_system_V01/Body_ECU/Interrupt to RPS1/Triggered Subsystem ==
  Interrupts : TriggerPort  VariantControl=(inherit)
  Add : Sum
  Constant : Constant  SampleTime=-1
  Data Store Read1 : DataStoreRead  DataStoreName=Count  IndexOptions=Index vector (dialog)  Indices=1  OutputSizes=1
  Data Store Write : DataStoreWrite  DataStoreName=Count  IndexOptions=Index vector (dialog)  Indices=1  OutputSizes=1
  RPS : Outport
  wires:
  Constant/1 -> Add/1
  Add/1 -> Data Store Write/1, RPS/1
  Data Store Read1/1 -> Add/2

== system Vehicle_model_with_controllers_in_continuous_system_V01/Body_ECU/Interrupt to RPS1/Triggered Subsystem1 ==
  Trigger : TriggerPort  VariantControl=(inherit)
  Constant : Constant  Value=0
  Data Store Write : DataStoreWrite  DataStoreName=Count  IndexOptions=Index vector (dialog)  Indices=1  OutputSizes=1
  wires:
  Constant/1 -> Data Store Write/1

== system Vehicle_model_with_controllers_in_continuous_system_V01/Vehicle_model/Car Plant Model/Electrical  ==
  Left_Ind_Status : Inport
  Right_Ind_Status : Inport  Port=2
  Lights : Subsystem
  Left_Indicator_light : Outport
  Right_Indicator_Light : Outport  Port=2
  wires:
  Left_Ind_Status/1 -> Lights/1(Left_Ind_Status)
  Right_Ind_Status/1 -> Lights/2(Right_Ind_Status)
  Lights/1(Left_Indicator_light) -> Left_Indicator_light/1
  Lights/2(Right_Indicator_Light) -> Right_Indicator_Light/1

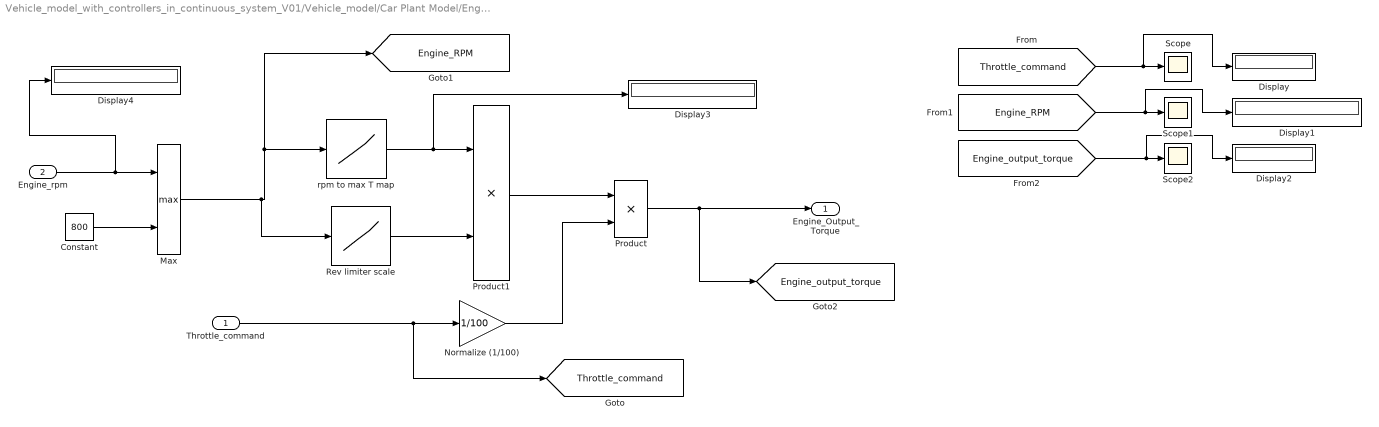
== system Vehicle_model_with_controllers_in_continuous_system_V01/Vehicle_model/Car Plant Model/Engine ==
  Throttle_command : Inport
  Engine_rpm : Inport  Port=2
  Constant : Constant  Value=800
  Display{,1..4} (5 alike) : Display
  Max : MinMax  Function=max  Inputs=2
  Normalize (1/100) : Gain  Gain=1/100
  Product : Product
  Product1 : Product
  Rev limiter scale : Lookup_n-D  NumberOfTableDimensions=1  BreakpointsForDimension1=[6200;6300;6400;6500;6600]  Table=[1;0.8;0.4;0.1;0]  ExtrapMethod=Clip  InternalRulePriority=Speed  RndMeth=Simplest
  Scope : Scope
      settings: DataLoggingVariableName=ScopeData13
  Scope1 : Scope
      settings: DataLoggingVariableName=ScopeData14
  Scope2 : Scope
      settings: DataLoggingVariableName=ScopeData15
  rpm to max T map : Lookup_n-D  NumberOfTableDimensions=1  BreakpointsForDimension1=[800;1500;2500;3500;4500;5500;6500]  Table=[90;180;240;250;235;190;120]  InternalRulePriority=Speed  RndMeth=Simplest
  Engine_Output_Torque : Outport
  tag scope: Engine_RPM=global, Engine_output_torque=global, Throttle_command=global
  wires:
  Throttle_command/1 -> Normalize (1/100)/1, [Throttle_command]
  Normalize (1/100)/1 -> Product/2
  rpm to max T map/1 -> Product1/1, Display3/1
  Product/1 -> Engine_Output_Torque/1, [Engine_output_torque]
  [Throttle_command] -> Display/1, Scope/1
  [Engine_RPM] -> Display1/1, Scope1/1
  [Engine_output_torque] -> Display2/1, Scope2/1
  Engine_rpm/1 -> Display4/1, Max/1
  Max/1 -> Rev limiter scale/1, [Engine_RPM], rpm to max T map/1
  Constant/1 -> Max/2
  Product1/1 -> Product/1
  Rev limiter scale/1 -> Product1/2

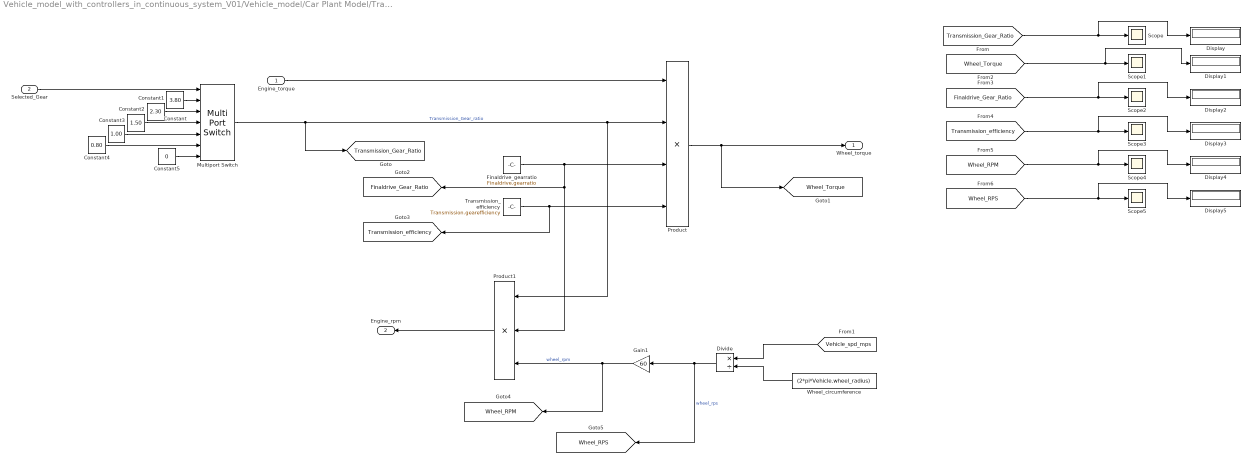
== system Vehicle_model_with_controllers_in_continuous_system_V01/Vehicle_model/Car Plant Model/Transmission ==
  Engine_torque : Inport
  Selected_Gear : Inport  Port=2
  Constant : Constant  Value=3.80
  Constant1 : Constant  Value=2.30
  Constant2 : Constant  Value=1.50
  Constant3 : Constant  Value=1.00
  Constant4 : Constant  Value=0.80
  Constant5 : Constant  Value=0
  Display{,1..5} (6 alike) : Display
  Divide : Product  Inputs=*/
  Finaldrive_gearratio : Constant  Value=Finaldrive.gearratio
  Gain1 : Gain  Gain=60
  Multiport Switch : MultiPortSwitch  Inputs=5  DataPortForDefault=Additional data port  DiagnosticForDefault=None  SaturateOnIntegerOverflow=off  InputSameDT=off
  Product : Product  Inputs=4
  Product1 : Product  Inputs=3
  Scope{,1..5} (6 alike) : Scope
      Scope settings: DataLoggingVariableName=ScopeData16
      Scope1 settings: ActiveDisplayYMinimum=234.61999999999989  ActiveDisplayYMaximum=2234.62  DataLoggingVariableName=ScopeData17
      Scope2 settings: DataLoggingVariableName=ScopeData18
      Scope3 settings: DataLoggingVariableName=ScopeData19
      Scope4 settings: DataLoggingVariableName=ScopeData20
      Scope5 settings: DataLoggingVariableName=ScopeData21
  Transmission_efficiency : Constant  Value=Transmission.gearefficiency
  Wheel_circumference : Constant  Value=(2*pi*Vehicle.wheel_radius)
  Wheel_torque : Outport
  Engine_rpm : Outport  Port=2
  tag scope: Finaldrive_Gear_Ratio=global, Transmission_Gear_Ratio=global, Transmission_efficiency=global, Wheel_RPM=global, Wheel_RPS=global, Wheel_Torque=global
  wires:
  Gain1/1 -> [Wheel_RPM], Product1/3  "wheel_rpm"
  [Vehicle_spd_mps] -> Divide/1
  Wheel_circumference/1 -> Divide/2
  Divide/1 -> [Wheel_RPS], Gain1/1  "wheel_rps"
  Constant/1 -> Multiport Switch/2
  Constant1/1 -> Multiport Switch/3
  Constant2/1 -> Multiport Switch/4
  Constant3/1 -> Multiport Switch/5
  Constant4/1 -> Multiport Switch/6
  Constant5/1 -> Multiport Switch/7
  Selected_Gear/1 -> Multiport Switch/1
  Product/1 -> [Wheel_Torque], Wheel_torque/1
  Engine_torque/1 -> Product/1
  Multiport Switch/1 -> [Transmission_Gear_Ratio], Product1/1, Product/2  "Transmission_Gear_ratio"
  Transmission_efficiency/1 -> [Transmission_efficiency], Product/4
  Product1/1 -> Engine_rpm/1
  Finaldrive_gearratio/1 -> Product1/2, [Finaldrive_Gear_Ratio], Product/3
  [Transmission_Gear_Ratio] -> Scope/1, Display/1
  [Wheel_Torque] -> Scope1/1, Display1/1
  [Finaldrive_Gear_Ratio] -> Scope2/1, Display2/1
  [Transmission_efficiency] -> Scope3/1, Display3/1
  [Wheel_RPM] -> Scope4/1, Display4/1
  [Wheel_RPS] -> Scope5/1, Display5/1

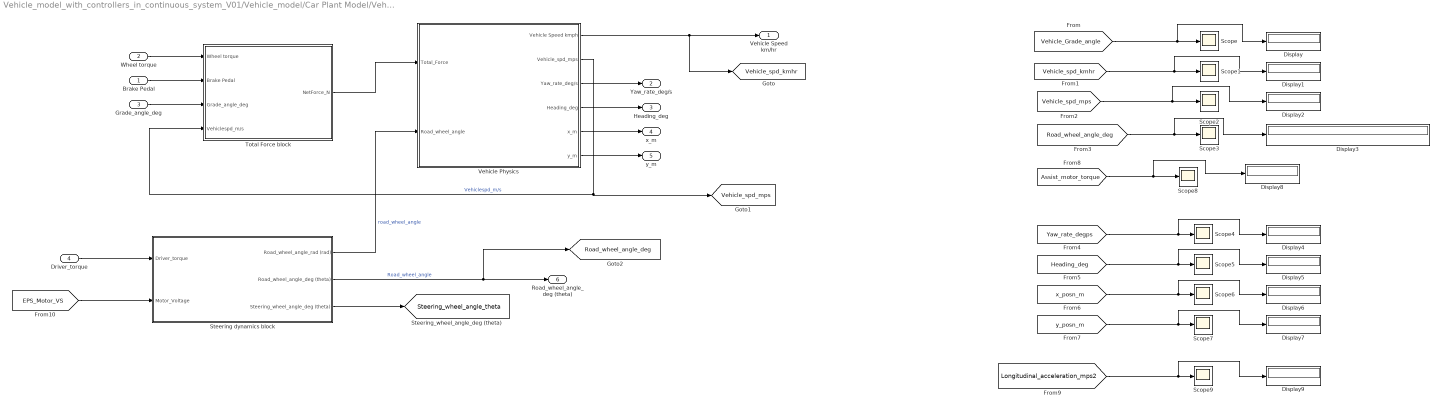
== system Vehicle_model_with_controllers_in_continuous_system_V01/Vehicle_model/Car Plant Model/Vehicle Dynamics ==
  Brake Pedal : Inport
  Wheel torque : Inport  Port=2
  Grade_angle_deg : Inport  Port=3
  Driver_torque : Inport  Port=4
  Display{,1..9} (10 alike) : Display
      Display3 settings: Format=long_e
  Scope{,1..9} (10 alike) : Scope
      Scope settings: DataLoggingVariableName=ScopeData22
      Scope1 settings: DataLoggingVariableName=ScopeData23
      Scope2 settings: DataLoggingVariableName=ScopeData24
      Scope3 settings: DataLoggingVariableName=ScopeData25
      Scope4 settings: DataLoggingVariableName=ScopeData26
      Scope5 settings: DataLoggingVariableName=ScopeData27
      Scope6 settings: DataLoggingVariableName=ScopeData28
      Scope7 settings: DataLoggingVariableName=ScopeData29
      Scope8 settings: DataLoggingVariableName=ScopeData33
      Scope9 settings: DataLoggingVariableName=ScopeData48
  Steering dynamics block : Subsystem
  Total Force block : Subsystem
  Vehicle Physics : Subsystem
  Vehicle Speed km/hr : Outport
  Yaw_rate_deg/s : Outport  Port=2
  Heading_deg : Outport  Port=3
  x_m : Outport  Port=4
  y_m : Outport  Port=5
  Road_wheel_angle_deg (theta) : Outport  Port=6
  tag scope: Road_wheel_angle_deg=global, Steering_wheel_angle_theta=global, Vehicle_spd_kmhr=global, Vehicle_spd_mps=global
  wires:
  Vehicle Physics/1(Vehicle Speed kmph) -> [Vehicle_spd_kmhr], Vehicle Speed km/hr/1
  Vehicle Physics/2(Vehicle_spd_mps) -> Total Force block/4(Vehiclespd_m/s), [Vehicle_spd_mps]  "Vehiclespd_m/s"
  Wheel torque/1 -> Total Force block/1(Wheel torque)
  Brake Pedal/1 -> Total Force block/2(Brake Pedal)
  Grade_angle_deg/1 -> Total Force block/3(Grade_angle_deg)
  Total Force block/1(NetForce_N) -> Vehicle Physics/1(Total_Force)
  Vehicle Physics/3(Yaw_rate_deg/s) -> Yaw_rate_deg/s/1
  Vehicle Physics/4(Heading_deg) -> Heading_deg/1
  Vehicle Physics/5(x_m) -> x_m/1
  Vehicle Physics/6(y_m) -> y_m/1
  Driver_torque/1 -> Steering dynamics block/1(Driver_torque)
  Steering dynamics block/1(Road_wheel_angle_rad (rad)) -> Vehicle Physics/2(Road_wheel_angle)  "road_wheel_angle"
  Steering dynamics block/3(Steering_wheel_angle_deg (theta)) -> [Steering_wheel_angle_theta]
  Steering dynamics block/2(Road_wheel_angle_deg (theta)) -> [Road_wheel_angle_deg], Road_wheel_angle_deg (theta)/1  "Road_wheel_angle"
  [Vehicle_Grade_angle] -> Display/1, Scope/1
  [Vehicle_spd_kmhr] -> Display1/1, Scope1/1
  [Vehicle_spd_mps] -> Display2/1, Scope2/1
  [Road_wheel_angle_deg] -> Display3/1, Scope3/1
  [Yaw_rate_degps] -> Display4/1, Scope4/1
  [Heading_deg] -> Display5/1, Scope5/1
  [x_posn_m] -> Display6/1, Scope6/1
  [y_posn_m] -> Display7/1, Scope7/1
  [Assist_motor_torque] -> Display8/1, Scope8/1
  [Longitudinal_acceleration_mps2] -> Display9/1, Scope9/1
  [EPS_Motor_VS] -> Steering dynamics block/2(Motor_Voltage)

== system Vehicle_model_with_controllers_in_continuous_system_V01/Vehicle_model/Driver//Controller_I_O/CONTROLLER_I_O ==
  Left_lndicator_status : Inport
  Right_Indicator_status : Inport  Port=2
  Controller_Accel_Cmd : Inport  Port=3
  EPS_Motor_Control : Inport  Port=4
  Body ECU : Subsystem
  Implement_ECU : Subsystem
  PT_ECU : Subsystem
  Left_lndicator_status_cmd : Outport
  Right_lndicator_status_cmd : Outport  Port=2
  Controller_Accelerator_Command : Outport  Port=3
  EPS_Motor_VS : Outport  Port=4
  wires:
  Left_lndicator_status/1 -> Body ECU/1(In1)
  Right_Indicator_status/1 -> Body ECU/2(In2)
  Body ECU/1(Out1) -> Left_lndicator_status_cmd/1
  Body ECU/2(Out2) -> Right_lndicator_status_cmd/1
  Controller_Accel_Cmd/1 -> PT_ECU/1(In1)
  PT_ECU/1(Out1) -> Controller_Accelerator_Command/1
  EPS_Motor_Control/1 -> Implement_ECU/1(In1)
  Implement_ECU/1(Out1) -> EPS_Motor_VS/1

== system Vehicle_model_with_controllers_in_continuous_system_V01/Vehicle_model/Driver//Controller_I_O/DRIVER I_O ==
  Driver_pedal : Inport
  Selected_Gear : Inport  Port=2
  Steering_wheel_angle_set : Inport  Port=3
  Steering_wheel_angle_output : Inport  Port=4
  Cruise ON/OFF switch : Inport  Port=5
  Cruise Setting : Inport  Port=6
  Drivepdl_interpretor : Subsystem
  Set_Gear : Subsystem
  Steering_wheel_angle to Driver_torque : Subsystem
  Subsystem : Subsystem
  Driver_Accelerator_pedal : Outport
  Driver_Brake_pedal : Outport  Port=2
  Gear_selected : Outport  Port=3
  Driver_steering_torque : Outport  Port=4
  Cruise Master SW : Outport  Port=5
  Cuise Setting : Outport  Port=6
  wires:
  Drivepdl_interpretor/2(Drvr_Brk_pdl) -> Driver_Brake_pedal/1
  Driver_pedal/1 -> Drivepdl_interpretor/1(Driver_pdl)
  Drivepdl_interpretor/1(Drve_Acc_pdl) -> Driver_Accelerator_pedal/1
  Steering_wheel_angle to Driver_torque/1(Driver_torque) -> Driver_steering_torque/1
  Selected_Gear/1 -> Set_Gear/1(In1)
  Steering_wheel_angle_set/1 -> Steering_wheel_angle to Driver_torque/1(desired angle)
  Set_Gear/1(Out1) -> Gear_selected/1
  Steering_wheel_angle_output/1 -> Steering_wheel_angle to Driver_torque/2(actual angle)
  Cruise Setting/1 -> Subsystem/2(In2)
  Cruise ON/OFF switch/1 -> Subsystem/1(In1)
  Subsystem/1(Out1) -> Cruise Master SW/1
  Subsystem/2(Out2) -> Cuise Setting/1

== system Vehicle_model_with_controllers_in_continuous_system_V01/Vehicle_model/SENSORS/DASHBOARD AND OTHER SENSORS//COMMUNICATION ==
  Display : Display
  Display1 : Display
  Display2 : Display
  Scope : Scope
      settings: DataLoggingVariableName=ScopeData53
  Scope1 : Scope
      settings: DataLoggingVariableName=ScopeData54
  Scope2 : Scope
      settings: DataLoggingVariableName=ScopeData8
  Out1 : Outport
  Out2 : Outport  Port=2
  Out3 : Outport  Port=3
  wires:
  [Cruise_setting] -> Display1/1, Scope1/1, Out2/1
  [Cruise_On_Off_SW] -> Display/1, Scope/1, Out1/1
  [Gear_selected] -> Display2/1, Scope2/1, Out3/1

== system Vehicle_model_with_controllers_in_continuous_system_V01/Vehicle_model/SENSORS/PEDAL SENSORS ==
  Display5 : Display
  Display6 : Display
  Scope1 : Scope
      settings: DataLoggingVariableName=ScopeData42
  Scope2 : Scope
      settings: DataLoggingVariableName=ScopeData43
  Out1 : Outport
  Out2 : Outport  Port=2
  wires:
  [Driver_Brake_Pedal] -> Display6/1, Out2/1, Scope2/1
  [Driver_Accelerator_Pedal] -> Out1/1, Scope1/1, Display5/1

== system Vehicle_model_with_controllers_in_continuous_system_V01/Vehicle_model/SENSORS/POWER TRAIN SENSORS ==
  Display{,1..3} (4 alike) : Display
  Scope{,1..3} (4 alike) : Scope
      Scope settings: DataLoggingVariableName=ScopeData46
      Scope1 settings: DataLoggingVariableName=ScopeData44
      Scope2 settings: DataLoggingVariableName=ScopeData45
      Scope3 settings: DataLoggingVariableName=ScopeData47
  Out1 : Outport
  Out2 : Outport  Port=2
  Out3 : Outport  Port=3
  Out4 : Outport  Port=4
  wires:
  [Engine_RPM] -> Out1/1, Display1/1, Scope1/1
  [Engine_output_torque] -> Scope2/1, Display2/1, Out2/1
  [Selected_Gear] -> Out3/1, Display/1, Scope/1
  [Wheel_Torque] -> Scope3/1, Out4/1, Display3/1

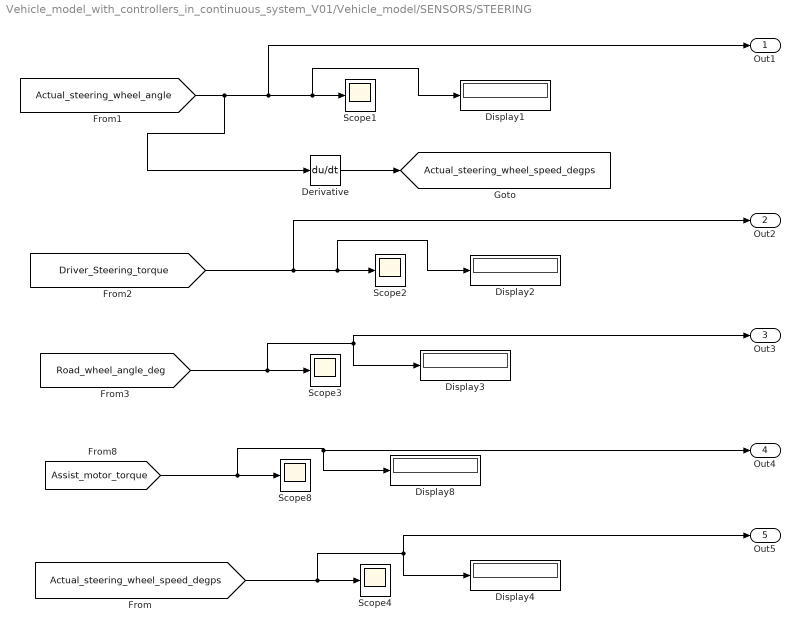
== system Vehicle_model_with_controllers_in_continuous_system_V01/Vehicle_model/SENSORS/STEERING ==
  Derivative : Derivative
  Display{1..4,8} (5 alike) : Display
  Scope{1..4,8} (5 alike) : Scope
      Scope1 settings: DataLoggingVariableName=ScopeData30
      Scope2 settings: DataLoggingVariableName=ScopeData31
      Scope3 settings: DataLoggingVariableName=ScopeData32
      Scope4 settings: DataLoggingVariableName=ScopeData35
      Scope8 settings: DataLoggingVariableName=ScopeData34
  Out1 : Outport
  Out2 : Outport  Port=2
  Out3 : Outport  Port=3
  Out4 : Outport  Port=4
  Out5 : Outport  Port=5
  tag scope: Actual_steering_wheel_speed_degps=global
  wires:
  [Driver_Steering_torque] -> Out2/1, Display2/1, Scope2/1
  [Road_wheel_angle_deg] -> Display3/1, Out3/1, Scope3/1
  [Assist_motor_torque] -> Out4/1, Display8/1, Scope8/1
  [Actual_steering_wheel_speed_degps] -> Out5/1, Display4/1, Scope4/1
  Derivative/1 -> [Actual_steering_wheel_speed_degps]
  [Actual_steering_wheel_angle] -> Derivative/1, Out1/1, Display1/1, Scope1/1

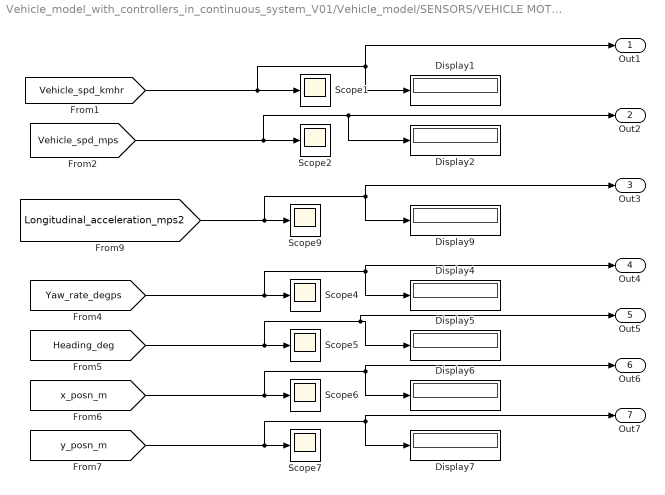
== system Vehicle_model_with_controllers_in_continuous_system_V01/Vehicle_model/SENSORS/VEHICLE MOTION SENSORS ==
  Display{1..2,4..7,9} (7 alike) : Display
  Scope{1..2,4..7,9} (7 alike) : Scope
      Scope1 settings: DataLoggingVariableName=ScopeData36
      Scope2 settings: DataLoggingVariableName=ScopeData37
      Scope4 settings: DataLoggingVariableName=ScopeData38
      Scope5 settings: DataLoggingVariableName=ScopeData39
      Scope6 settings: DataLoggingVariableName=ScopeData40
      Scope7 settings: DataLoggingVariableName=ScopeData41
      Scope9 settings: DataLoggingVariableName=ScopeData49
  Out1 : Outport
  Out2 : Outport  Port=2
  Out3 : Outport  Port=3
  Out4 : Outport  Port=4
  Out5 : Outport  Port=5
  Out6 : Outport  Port=6
  Out7 : Outport  Port=7
  wires:
  [Vehicle_spd_kmhr] -> Display1/1, Out1/1, Scope1/1
  [Vehicle_spd_mps] -> Out2/1, Display2/1, Scope2/1
  [Yaw_rate_degps] -> Display4/1, Out4/1, Scope4/1
  [Heading_deg] -> Out5/1, Display5/1, Scope5/1
  [y_posn_m] -> Display7/1, Out7/1, Scope7/1
  [x_posn_m] -> Display6/1, Out6/1, Scope6/1
  [Longitudinal_acceleration_mps2] -> Display9/1, Out3/1, Scope9/1

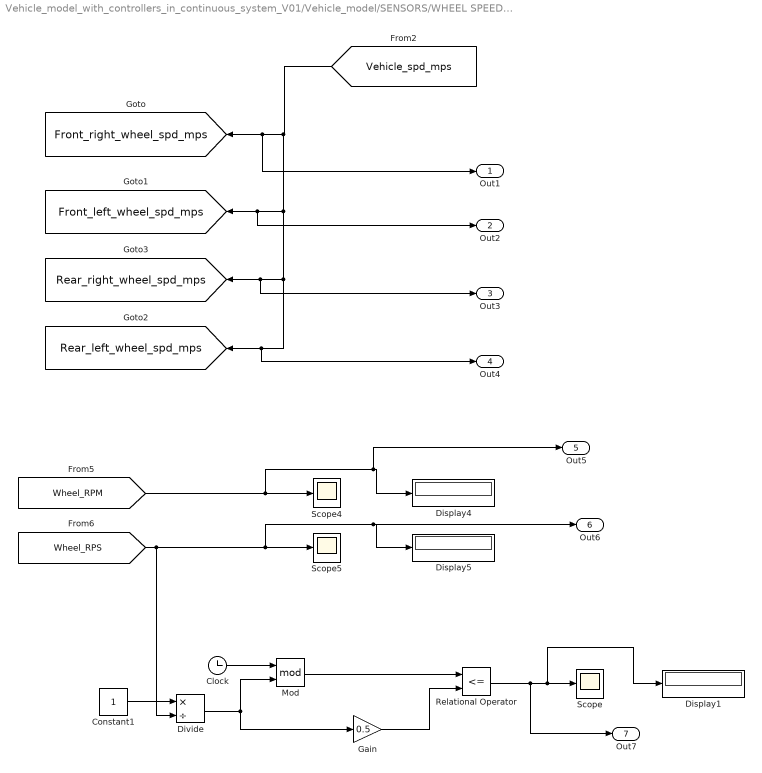
== system Vehicle_model_with_controllers_in_continuous_system_V01/Vehicle_model/SENSORS/WHEEL SPEED SENSORS ==
  Clock : Clock
  Constant1 : Constant
  Display1 : Display
  Display4 : Display
  Display5 : Display
  Divide : Product  Inputs=*/
  Gain : Gain  Gain=0.5
  Mod : Math  Operator=mod
  Relational Operator : RelationalOperator  Operator=<=  OutDataTypeStr=boolean  RndMeth=Simplest  InputSameDT=off
  Scope : Scope
      settings: ActiveDisplayYMinimum=-0.12499999999999997  ActiveDisplayYMaximum=1.125  DataLoggingVariableName=ScopeData52
  Scope4 : Scope
      settings: ActiveDisplayYMinimum=948.95105383066675  ActiveDisplayYMaximum=1094.4080240648523  DataLoggingVariableName=ScopeData50
  Scope5 : Scope
      settings: ActiveDisplayYMinimum=15.81585089717778  ActiveDisplayYMaximum=18.2401337344142  DataLoggingVariableName=ScopeData51
  Out1 : Outport
  Out2 : Outport  Port=2
  Out3 : Outport  Port=3
  Out4 : Outport  Port=4
  Out5 : Outport  Port=5
  Out6 : Outport  Port=6
  Out7 : Outport  Port=7
  tag scope: Front_left_wheel_spd_mps=global, Front_right_wheel_spd_mps=global, Rear_left_wheel_spd_mps=global, Rear_right_wheel_spd_mps=global
  wires:
  [Vehicle_spd_mps] -> Out4/1, [Rear_left_wheel_spd_mps], Out3/1, [Rear_right_wheel_spd_mps], Out2/1, [Front_left_wheel_spd_mps], Out1/1, [Front_right_wheel_spd_mps]
  [Wheel_RPS] -> Divide/2, Scope5/1, Out6/1, Display5/1
  [Wheel_RPM] -> Scope4/1, Out5/1, Display4/1
  Clock/1 -> Mod/1
  Gain/1 -> Relational Operator/2
  Relational Operator/1 -> Out7/1, Display1/1, Scope/1
  Constant1/1 -> Divide/1
  Divide/1 -> Gain/1, Mod/2
  Mod/1 -> Relational Operator/1

== system Vehicle_model_with_controllers_in_continuous_system_V01/Vehicle_model/Car Plant Model/Electrical /Lights ==
  Left_Ind_Status : Inport
  Right_Ind_Status : Inport  Port=2
  Constant : Constant
  Constant1 : Constant  Value=0
  Constant2 : Constant
  Constant3 : Constant  Value=0
  Switch : Switch  Criteria=u2 > Threshold  SaturateOnIntegerOverflow=off  InputSameDT=off
  Switch1 : Switch  Criteria=u2 > Threshold  SaturateOnIntegerOverflow=off  InputSameDT=off
  Left_Indicator_light : Outport
  Right_Indicator_Light : Outport  Port=2
  wires:
  Constant/1 -> Switch/1
  Left_Ind_Status/1 -> Switch/2
  Switch/1 -> Left_Indicator_light/1
  Constant1/1 -> Switch/3
  Constant2/1 -> Switch1/1
  Switch1/1 -> Right_Indicator_Light/1
  Right_Ind_Status/1 -> Switch1/2
  Constant3/1 -> Switch1/3
